simulink model "SimplePengulumSystem"  (R2024a)
settings: Solver=ode45  StartTime=0.0  StopTime=10.0  RelTol=1e-10
settings Model: Creator=tristan  LastModifiedBy=tristan

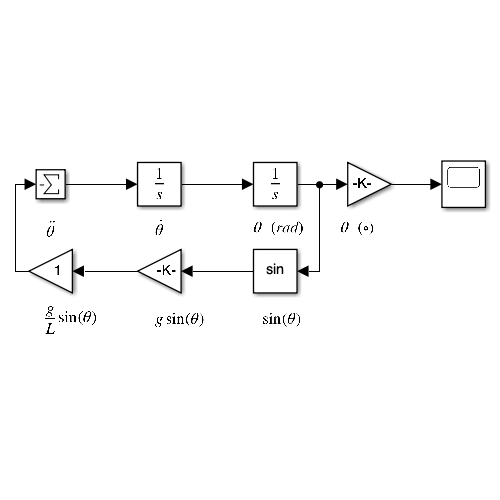
[thumbnail: Simulink's stored preview of the top-level diagram]
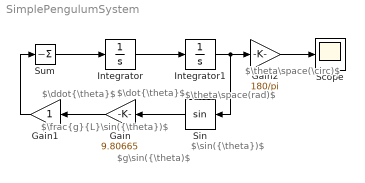
== system SimplePengulumSystem ==
  note: $\dot{\theta}$
  note: $\ddot{\theta}$
  note: $\theta\space(rad)$
  note: $g\sin({\theta)$
  note: $\frac{g}{L}\sin({\theta})$
  note: $\sin({\theta})$
  note: $\theta\space(\circ)$
  Gain : Gain  Gain=9.80665
  Gain1 : Gain
  Gain2 : Gain  Gain=180/pi
  Integrator : Integrator
  Integrator1 : Integrator  InitialCondition=pi/6
  Scope : Scope
  Sin : Trigonometry
  Sum : Sum  Inputs=-
  wires:
  Sum/1 -> Integrator/1
  Integrator/1 -> Integrator1/1
  Gain/1 -> Gain1/1
  Integrator1/1 -> Gain2/1, Sin/1
  Sin/1 -> Gain/1
  Gain1/1 -> Sum/1
  Gain2/1 -> Scope/1
